simulink model "gm_soc_dvbs2_fpga"  (R2025b)
settings: Solver=VariableStepAuto  StartTime=0.0  StopTime=10.0  RelTol=1e-3
InitFcn:
  | soc_dvbs2_init;
undefined symbols (not defined in the file or in its folder): Add, coefficientsLog, coefficientsSqrt1, coefficientsSqrt2, dataBits, Deinterleaver, designMultirateFIR, noisePow, Shift, Short, soc_dvbs2_designFIRFilter, soc_dvbs2_txPacketBits, syncWord, txDataOut, txFiltCoeff, XData
libraries: simulink x304, hdlsllib x265, dspsigops x15, dsphdlfiltering2 x8, hdlmdlgenlib x6, dsphdlsigops2 x5, commseqgen3 x5, dsphdlmathfun2 x3, hwlogicconnlib x2, whdledac x2, commhdlcrc x2, whdlutilities x1
(part 28 of 36)

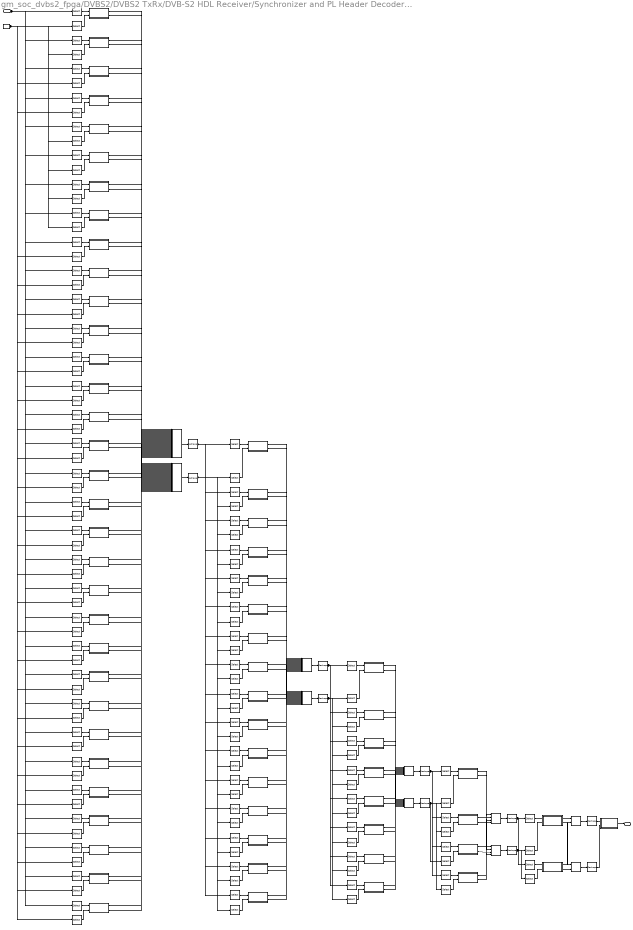
== system gm_soc_dvbs2_fpga/DVBS2/DVBS2 TxRx/DVB-S2 HDL Receiver/Synchronizer and PL Header Decoder/PL Header Recovery/PL Header Decoder/ML Decoder/Get Min Index ==
  dataIn : Inport  OutDataTypeStr=fixdt(1, 25, 15)  PortDimensions=[64]  SampleTime=2.5e-07
  For Each Subsystem1_instance1 : Subsystem
  For Each Subsystem1_instance10 : Subsystem
  For Each Subsystem1_instance11 : Subsystem
  For Each Subsystem1_instance12 : Subsystem
  For Each Subsystem1_instance13 : Subsystem
  For Each Subsystem1_instance14 : Subsystem
  For Each Subsystem1_instance15 : Subsystem
  For Each Subsystem1_instance16 : Subsystem
  For Each Subsystem1_instance2 : Subsystem
  For Each Subsystem1_instance3 : Subsystem
  For Each Subsystem1_instance4 : Subsystem
  For Each Subsystem1_instance5 : Subsystem
  For Each Subsystem1_instance6 : Subsystem
  For Each Subsystem1_instance7 : Subsystem
  For Each Subsystem1_instance8 : Subsystem
  For Each Subsystem1_instance9 : Subsystem
  For Each Subsystem2_instance1 : Subsystem
  For Each Subsystem2_instance2 : Subsystem
  For Each Subsystem2_instance3 : Subsystem
  For Each Subsystem2_instance4 : Subsystem
  For Each Subsystem2_instance5 : Subsystem
  For Each Subsystem2_instance6 : Subsystem
  For Each Subsystem2_instance7 : Subsystem
  For Each Subsystem2_instance8 : Subsystem
  For Each Subsystem3_instance1 : Subsystem
  For Each Subsystem3_instance2 : Subsystem
  For Each Subsystem3_instance3 : Subsystem
  For Each Subsystem3_instance4 : Subsystem
  For Each Subsystem4_instance1 : Subsystem
  For Each Subsystem4_instance2 : Subsystem
  For Each Subsystem5 : Subsystem
  For Each Subsystem_instance1 : Subsystem
  For Each Subsystem_instance10 : Subsystem
  For Each Subsystem_instance11 : Subsystem
  For Each Subsystem_instance12 : Subsystem
  For Each Subsystem_instance13 : Subsystem
  For Each Subsystem_instance14 : Subsystem
  For Each Subsystem_instance15 : Subsystem
  For Each Subsystem_instance16 : Subsystem
  For Each Subsystem_instance17 : Subsystem
  For Each Subsystem_instance18 : Subsystem
  For Each Subsystem_instance19 : Subsystem
  For Each Subsystem_instance2 : Subsystem
  For Each Subsystem_instance20 : Subsystem
  For Each Subsystem_instance21 : Subsystem
  For Each Subsystem_instance22 : Subsystem
  For Each Subsystem_instance23 : Subsystem
  For Each Subsystem_instance24 : Subsystem
  For Each Subsystem_instance25 : Subsystem
  For Each Subsystem_instance26 : Subsystem
  For Each Subsystem_instance27 : Subsystem
  For Each Subsystem_instance28 : Subsystem
  For Each Subsystem_instance29 : Subsystem
  For Each Subsystem_instance3 : Subsystem
  For Each Subsystem_instance30 : Subsystem
  For Each Subsystem_instance31 : Subsystem
  For Each Subsystem_instance32 : Subsystem
  For Each Subsystem_instance4 : Subsystem
  For Each Subsystem_instance5 : Subsystem
  For Each Subsystem_instance6 : Subsystem
  For Each Subsystem_instance7 : Subsystem
  For Each Subsystem_instance8 : Subsystem
  For Each Subsystem_instance9 : Subsystem
  Selector_1 : Selector  InputPortWidth=64  IndexOptions=Index vector (dialog)  Indices=double([1 2])  OutputSizes=1
  Selector_10 : Selector  InputPortWidth=64  IndexOptions=Index vector (dialog)  Indices=double([19 20])  OutputSizes=1
  Selector_101 : Selector  InputPortWidth=64  IndexOptions=Index vector (dialog)  Indices=double([19 20])  OutputSizes=1
  Selector_102 : Selector  InputPortWidth=32  IndexOptions=Index vector (dialog)  Indices=double([19 20])  OutputSizes=1
  Selector_103 : Selector  InputPortWidth=32  IndexOptions=Index vector (dialog)  Indices=double([19 20])  OutputSizes=1
  Selector_11 : Selector  InputPortWidth=64  IndexOptions=Index vector (dialog)  Indices=double([21 22])  OutputSizes=1
  Selector_110 : Selector  InputPortWidth=64  IndexOptions=Index vector (dialog)  Indices=double([1 2])  OutputSizes=1
  Selector_111 : Selector  InputPortWidth=64  IndexOptions=Index vector (dialog)  Indices=double([21 22])  OutputSizes=1
  Selector_112 : Selector  InputPortWidth=32  IndexOptions=Index vector (dialog)  Indices=double([1 2])  OutputSizes=1
  Selector_113 : Selector  InputPortWidth=32  IndexOptions=Index vector (dialog)  Indices=double([21 22])  OutputSizes=1
  Selector_114 : Selector  InputPortWidth=32  IndexOptions=Index vector (dialog)  Indices=double([1 2])  OutputSizes=1
  Selector_115 : Selector  InputPortWidth=32  IndexOptions=Index vector (dialog)  Indices=double([21 22])  OutputSizes=1
  Selector_116 : Selector  InputPortWidth=16  IndexOptions=Index vector (dialog)  Indices=double([1 2])  OutputSizes=1
  Selector_117 : Selector  InputPortWidth=16  IndexOptions=Index vector (dialog)  Indices=double([1 2])  OutputSizes=1
  Selector_118 : Selector  InputPortWidth=8  IndexOptions=Index vector (dialog)  Indices=double([1 2])  OutputSizes=1
  Selector_119 : Selector  InputPortWidth=8  IndexOptions=Index vector (dialog)  Indices=double([1 2])  OutputSizes=1
  Selector_12 : Selector  InputPortWidth=64  IndexOptions=Index vector (dialog)  Indices=double([23 24])  OutputSizes=1
  Selector_120 : Selector  InputPortWidth=4  IndexOptions=Index vector (dialog)  Indices=double([1 2])  OutputSizes=1
  Selector_121 : Selector  InputPortWidth=64  IndexOptions=Index vector (dialog)  Indices=double([23 24])  OutputSizes=1
  Selector_122 : Selector  InputPortWidth=32  IndexOptions=Index vector (dialog)  Indices=double([23 24])  OutputSizes=1
  Selector_123 : Selector  InputPortWidth=32  IndexOptions=Index vector (dialog)  Indices=double([23 24])  OutputSizes=1
  Selector_124 : Selector  InputPortWidth=4  IndexOptions=Index vector (dialog)  Indices=double([1 2])  OutputSizes=1
  Selector_13 : Selector  InputPortWidth=64  IndexOptions=Index vector (dialog)  Indices=double([25 26])  OutputSizes=1
  Selector_131 : Selector  InputPortWidth=64  IndexOptions=Index vector (dialog)  Indices=double([25 26])  OutputSizes=1
  Selector_132 : Selector  InputPortWidth=32  IndexOptions=Index vector (dialog)  Indices=double([25 26])  OutputSizes=1
  Selector_133 : Selector  InputPortWidth=32  IndexOptions=Index vector (dialog)  Indices=double([25 26])  OutputSizes=1
  Selector_14 : Selector  InputPortWidth=64  IndexOptions=Index vector (dialog)  Indices=double([27 28])  OutputSizes=1
  Selector_141 : Selector  InputPortWidth=64  IndexOptions=Index vector (dialog)  Indices=double([27 28])  OutputSizes=1
  Selector_142 : Selector  InputPortWidth=32  IndexOptions=Index vector (dialog)  Indices=double([27 28])  OutputSizes=1
  Selector_143 : Selector  InputPortWidth=32  IndexOptions=Index vector (dialog)  Indices=double([27 28])  OutputSizes=1
  Selector_15 : Selector  InputPortWidth=64  IndexOptions=Index vector (dialog)  Indices=double([29 30])  OutputSizes=1
  Selector_151 : Selector  InputPortWidth=64  IndexOptions=Index vector (dialog)  Indices=double([29 30])  OutputSizes=1
  Selector_152 : Selector  InputPortWidth=32  IndexOptions=Index vector (dialog)  Indices=double([29 30])  OutputSizes=1
  Selector_153 : Selector  InputPortWidth=32  IndexOptions=Index vector (dialog)  Indices=double([29 30])  OutputSizes=1
  Selector_16 : Selector  InputPortWidth=64  IndexOptions=Index vector (dialog)  Indices=double([31 32])  OutputSizes=1
  Selector_161 : Selector  InputPortWidth=64  IndexOptions=Index vector (dialog)  Indices=double([31 32])  OutputSizes=1
  Selector_162 : Selector  InputPortWidth=32  IndexOptions=Index vector (dialog)  Indices=double([31 32])  OutputSizes=1
  Selector_163 : Selector  InputPortWidth=32  IndexOptions=Index vector (dialog)  Indices=double([31 32])  OutputSizes=1
  Selector_17 : Selector  InputPortWidth=64  IndexOptions=Index vector (dialog)  Indices=double([33 34])  OutputSizes=1
  Selector_171 : Selector  InputPortWidth=64  IndexOptions=Index vector (dialog)  Indices=double([33 34])  OutputSizes=1
  Selector_18 : Selector  InputPortWidth=64  IndexOptions=Index vector (dialog)  Indices=double([35 36])  OutputSizes=1
  Selector_181 : Selector  InputPortWidth=64  IndexOptions=Index vector (dialog)  Indices=double([35 36])  OutputSizes=1
  Selector_19 : Selector  InputPortWidth=64  IndexOptions=Index vector (dialog)  Indices=double([37 38])  OutputSizes=1
  Selector_191 : Selector  InputPortWidth=64  IndexOptions=Index vector (dialog)  Indices=double([37 38])  OutputSizes=1
  Selector_2 : Selector  InputPortWidth=64  IndexOptions=Index vector (dialog)  Indices=double([3 4])  OutputSizes=1
  Selector_20 : Selector  InputPortWidth=64  IndexOptions=Index vector (dialog)  Indices=double([39 40])  OutputSizes=1
  Selector_201 : Selector  InputPortWidth=64  IndexOptions=Index vector (dialog)  Indices=double([39 40])  OutputSizes=1
  Selector_21 : Selector  InputPortWidth=64  IndexOptions=Index vector (dialog)  Indices=double([41 42])  OutputSizes=1
  Selector_210 : Selector  InputPortWidth=64  IndexOptions=Index vector (dialog)  Indices=double([3 4])  OutputSizes=1
  Selector_211 : Selector  InputPortWidth=64  IndexOptions=Index vector (dialog)  Indices=double([41 42])  OutputSizes=1
  Selector_212 : Selector  InputPortWidth=32  IndexOptions=Index vector (dialog)  Indices=double([3 4])  OutputSizes=1
  Selector_213 : Selector  InputPortWidth=32  IndexOptions=Index vector (dialog)  Indices=double([3 4])  OutputSizes=1
  Selector_214 : Selector  InputPortWidth=16  IndexOptions=Index vector (dialog)  Indices=double([3 4])  OutputSizes=1
  Selector_215 : Selector  InputPortWidth=16  IndexOptions=Index vector (dialog)  Indices=double([3 4])  OutputSizes=1
  Selector_216 : Selector  InputPortWidth=8  IndexOptions=Index vector (dialog)  Indices=double([3 4])  OutputSizes=1
  Selector_217 : Selector  InputPortWidth=8  IndexOptions=Index vector (dialog)  Indices=double([3 4])  OutputSizes=1
  Selector_218 : Selector  InputPortWidth=4  IndexOptions=Index vector (dialog)  Indices=double([3 4])  OutputSizes=1
  Selector_219 : Selector  InputPortWidth=4  IndexOptions=Index vector (dialog)  Indices=double([3 4])  OutputSizes=1
  Selector_22 : Selector  InputPortWidth=64  IndexOptions=Index vector (dialog)  Indices=double([43 44])  OutputSizes=1
  Selector_221 : Selector  InputPortWidth=64  IndexOptions=Index vector (dialog)  Indices=double([43 44])  OutputSizes=1
  Selector_23 : Selector  InputPortWidth=64  IndexOptions=Index vector (dialog)  Indices=double([45 46])  OutputSizes=1
  Selector_231 : Selector  InputPortWidth=64  IndexOptions=Index vector (dialog)  Indices=double([45 46])  OutputSizes=1
  Selector_24 : Selector  InputPortWidth=64  IndexOptions=Index vector (dialog)  Indices=double([47 48])  OutputSizes=1
  Selector_241 : Selector  InputPortWidth=64  IndexOptions=Index vector (dialog)  Indices=double([47 48])  OutputSizes=1
  Selector_25 : Selector  InputPortWidth=64  IndexOptions=Index vector (dialog)  Indices=double([49 50])  OutputSizes=1
  Selector_251 : Selector  InputPortWidth=64  IndexOptions=Index vector (dialog)  Indices=double([49 50])  OutputSizes=1
  Selector_26 : Selector  InputPortWidth=64  IndexOptions=Index vector (dialog)  Indices=double([51 52])  OutputSizes=1
  Selector_261 : Selector  InputPortWidth=64  IndexOptions=Index vector (dialog)  Indices=double([51 52])  OutputSizes=1
  Selector_27 : Selector  InputPortWidth=64  IndexOptions=Index vector (dialog)  Indices=double([53 54])  OutputSizes=1
  Selector_271 : Selector  InputPortWidth=64  IndexOptions=Index vector (dialog)  Indices=double([53 54])  OutputSizes=1
  Selector_28 : Selector  InputPortWidth=64  IndexOptions=Index vector (dialog)  Indices=double([55 56])  OutputSizes=1
  Selector_281 : Selector  InputPortWidth=64  IndexOptions=Index vector (dialog)  Indices=double([55 56])  OutputSizes=1
  Selector_29 : Selector  InputPortWidth=64  IndexOptions=Index vector (dialog)  Indices=double([57 58])  OutputSizes=1
  Selector_291 : Selector  InputPortWidth=64  IndexOptions=Index vector (dialog)  Indices=double([57 58])  OutputSizes=1
  Selector_3 : Selector  InputPortWidth=64  IndexOptions=Index vector (dialog)  Indices=double([5 6])  OutputSizes=1
  Selector_30 : Selector  InputPortWidth=64  IndexOptions=Index vector (dialog)  Indices=double([59 60])  OutputSizes=1
  Selector_301 : Selector  InputPortWidth=64  IndexOptions=Index vector (dialog)  Indices=double([59 60])  OutputSizes=1
  Selector_31 : Selector  InputPortWidth=64  IndexOptions=Index vector (dialog)  Indices=double([61 62])  OutputSizes=1
  Selector_311 : Selector  InputPortWidth=64  IndexOptions=Index vector (dialog)  Indices=double([61 62])  OutputSizes=1
  Selector_32 : Selector  InputPortWidth=64  IndexOptions=Index vector (dialog)  Indices=double([63 64])  OutputSizes=1
  Selector_321 : Selector  InputPortWidth=64  IndexOptions=Index vector (dialog)  Indices=double([63 64])  OutputSizes=1
  Selector_33 : Selector  InputPortWidth=64  IndexOptions=Index vector (dialog)  Indices=double([5 6])  OutputSizes=1
  Selector_34 : Selector  InputPortWidth=32  IndexOptions=Index vector (dialog)  Indices=double([5 6])  OutputSizes=1
  Selector_35 : Selector  InputPortWidth=32  IndexOptions=Index vector (dialog)  Indices=double([5 6])  OutputSizes=1
  Selector_36 : Selector  InputPortWidth=16  IndexOptions=Index vector (dialog)  Indices=double([5 6])  OutputSizes=1
  Selector_37 : Selector  InputPortWidth=16  IndexOptions=Index vector (dialog)  Indices=double([5 6])  OutputSizes=1
  Selector_38 : Selector  InputPortWidth=8  IndexOptions=Index vector (dialog)  Indices=double([5 6])  OutputSizes=1
  Selector_39 : Selector  InputPortWidth=8  IndexOptions=Index vector (dialog)  Indices=double([5 6])  OutputSizes=1
  Selector_4 : Selector  InputPortWidth=64  IndexOptions=Index vector (dialog)  Indices=double([7 8])  OutputSizes=1
  Selector_41 : Selector  InputPortWidth=64  IndexOptions=Index vector (dialog)  Indices=double([7 8])  OutputSizes=1
  Selector_42 : Selector  InputPortWidth=32  IndexOptions=Index vector (dialog)  Indices=double([7 8])  OutputSizes=1
  Selector_43 : Selector  InputPortWidth=32  IndexOptions=Index vector (dialog)  Indices=double([7 8])  OutputSizes=1
  Selector_44 : Selector  InputPortWidth=16  IndexOptions=Index vector (dialog)  Indices=double([7 8])  OutputSizes=1
  Selector_45 : Selector  InputPortWidth=16  IndexOptions=Index vector (dialog)  Indices=double([7 8])  OutputSizes=1
  Selector_46 : Selector  InputPortWidth=8  IndexOptions=Index vector (dialog)  Indices=double([7 8])  OutputSizes=1
  Selector_47 : Selector  InputPortWidth=8  IndexOptions=Index vector (dialog)  Indices=double([7 8])  OutputSizes=1
  Selector_5 : Selector  InputPortWidth=64  IndexOptions=Index vector (dialog)  Indices=double([9 10])  OutputSizes=1
  Selector_51 : Selector  InputPortWidth=64  IndexOptions=Index vector (dialog)  Indices=double([9 10])  OutputSizes=1
  Selector_52 : Selector  InputPortWidth=32  IndexOptions=Index vector (dialog)  Indices=double([9 10])  OutputSizes=1
  Selector_53 : Selector  InputPortWidth=32  IndexOptions=Index vector (dialog)  Indices=double([9 10])  OutputSizes=1
  Selector_54 : Selector  InputPortWidth=16  IndexOptions=Index vector (dialog)  Indices=double([9 10])  OutputSizes=1
  Selector_55 : Selector  InputPortWidth=16  IndexOptions=Index vector (dialog)  Indices=double([9 10])  OutputSizes=1
  Selector_6 : Selector  InputPortWidth=64  IndexOptions=Index vector (dialog)  Indices=double([11 12])  OutputSizes=1
  Selector_61 : Selector  InputPortWidth=64  IndexOptions=Index vector (dialog)  Indices=double([11 12])  OutputSizes=1
  Selector_62 : Selector  InputPortWidth=32  IndexOptions=Index vector (dialog)  Indices=double([11 12])  OutputSizes=1
  Selector_63 : Selector  InputPortWidth=32  IndexOptions=Index vector (dialog)  Indices=double([11 12])  OutputSizes=1
  Selector_64 : Selector  InputPortWidth=16  IndexOptions=Index vector (dialog)  Indices=double([11 12])  OutputSizes=1
  Selector_65 : Selector  InputPortWidth=16  IndexOptions=Index vector (dialog)  Indices=double([11 12])  OutputSizes=1
  Selector_7 : Selector  InputPortWidth=64  IndexOptions=Index vector (dialog)  Indices=double([13 14])  OutputSizes=1
  Selector_71 : Selector  InputPortWidth=64  IndexOptions=Index vector (dialog)  Indices=double([13 14])  OutputSizes=1
  Selector_72 : Selector  InputPortWidth=32  IndexOptions=Index vector (dialog)  Indices=double([13 14])  OutputSizes=1
  Selector_73 : Selector  InputPortWidth=32  IndexOptions=Index vector (dialog)  Indices=double([13 14])  OutputSizes=1
  Selector_74 : Selector  InputPortWidth=16  IndexOptions=Index vector (dialog)  Indices=double([13 14])  OutputSizes=1
  Selector_75 : Selector  InputPortWidth=16  IndexOptions=Index vector (dialog)  Indices=double([13 14])  OutputSizes=1
  Selector_8 : Selector  InputPortWidth=64  IndexOptions=Index vector (dialog)  Indices=double([15 16])  OutputSizes=1
  Selector_81 : Selector  InputPortWidth=64  IndexOptions=Index vector (dialog)  Indices=double([15 16])  OutputSizes=1
  Selector_82 : Selector  InputPortWidth=32  IndexOptions=Index vector (dialog)  Indices=double([15 16])  OutputSizes=1
  Selector_83 : Selector  InputPortWidth=32  IndexOptions=Index vector (dialog)  Indices=double([15 16])  OutputSizes=1
  Selector_84 : Selector  InputPortWidth=16  IndexOptions=Index vector (dialog)  Indices=double([15 16])  OutputSizes=1
  Selector_85 : Selector  InputPortWidth=16  IndexOptions=Index vector (dialog)  Indices=double([15 16])  OutputSizes=1
  Selector_9 : Selector  InputPortWidth=64  IndexOptions=Index vector (dialog)  Indices=double([17 18])  OutputSizes=1
  Selector_91 : Selector  InputPortWidth=64  IndexOptions=Index vector (dialog)  Indices=double([17 18])  OutputSizes=1
  Selector_92 : Selector  InputPortWidth=32  IndexOptions=Index vector (dialog)  Indices=double([17 18])  OutputSizes=1
  Selector_93 : Selector  InputPortWidth=32  IndexOptions=Index vector (dialog)  Indices=double([17 18])  OutputSizes=1
  concatenate : Concatenate  NumInputs=32
  concatenate1 : Concatenate  NumInputs=32
  concatenate2 : Concatenate  NumInputs=16
  concatenate3 : Concatenate  NumInputs=16
  concatenate4 : Concatenate  NumInputs=8
  concatenate5 : Concatenate  NumInputs=8
  concatenate6 : Concatenate  NumInputs=4
  concatenate7 : Concatenate  NumInputs=4
  concatenate8 : Concatenate
  concatenate9 : Concatenate
  indices : Constant  Value=(0:63).'  OutDataTypeStr=fixdt(0,6,0)  SampleTime=-1
  t{,1..9} (10 alike) : Reshape
  out : Outport  SampleTime=2.5e-07
  wires:
  For Each Subsystem5/1(idxOut) -> out/1
  Selector_75/1 -> For Each Subsystem2_instance7/2(idxIn)
  Selector_39/1 -> For Each Subsystem3_instance3/2(idxIn)
  indices/1 -> Selector_311/1, Selector_271/1, Selector_261/1, Selector_251/1, Selector_241/1, Selector_231/1, Selector_211/1, Selector_181/1, Selector_171/1, Selector_131/1, Selector_101/1, Selector_81/1, Selector_61/1, Selector_41/1, Selector_33/1, Selector_210/1, Selector_110/1, Selector_281/1, Selector_161/1, Selector_301/1, Selector_91/1, Selector_151/1, Selector_191/1, Selector_291/1, Selector_121/1, Selector_321/1, Selector_51/1, Selector_111/1, Selector_221/1, Selector_201/1, Selector_71/1, Selector_141/1
  For Each Subsystem2_instance5/1(ValueOut) -> concatenate4/5
  For Each Subsystem2_instance6/1(ValueOut) -> concatenate4/6
  Selector_191/1 -> For Each Subsystem_instance19/2(idxIn)
  For Each Subsystem2_instance3/1(ValueOut) -> concatenate4/3
  Selector_35/1 -> For Each Subsystem1_instance3/2(idxIn)
  For Each Subsystem4_instance2/2(idxOut) -> concatenate9/2
  For Each Subsystem2_instance7/2(idxOut) -> concatenate5/7
  For Each Subsystem3_instance4/1(ValueOut) -> concatenate6/4
  For Each Subsystem2_instance1/2(idxOut) -> concatenate5/1
  For Each Subsystem_instance17/1(ValueOut) -> concatenate/17
  concatenate9/1 -> t9/1
  Selector_118/1 -> For Each Subsystem3_instance1/1(valueIn)
  Selector_16/1 -> For Each Subsystem_instance16/1(valueIn)
  For Each Subsystem3_instance2/2(idxOut) -> concatenate7/2
  Selector_1/1 -> For Each Subsystem_instance1/1(valueIn)
  Selector_74/1 -> For Each Subsystem2_instance7/1(valueIn)
  For Each Subsystem1_instance16/2(idxOut) -> concatenate3/16
  Selector_53/1 -> For Each Subsystem1_instance5/2(idxIn)
  Selector_291/1 -> For Each Subsystem_instance29/2(idxIn)
  For Each Subsystem2_instance3/2(idxOut) -> concatenate5/3
  Selector_17/1 -> For Each Subsystem_instance17/1(valueIn)
  concatenate7/1 -> t7/1
  For Each Subsystem4_instance2/1(ValueOut) -> concatenate8/2
  Selector_55/1 -> For Each Subsystem2_instance5/2(idxIn)
  t1/1 -> Selector_163/1, Selector_153/1, Selector_143/1, Selector_123/1, Selector_103/1, Selector_93/1, Selector_83/1, Selector_73/1, Selector_63/1, Selector_53/1, Selector_213/1, Selector_114/1, Selector_133/1, Selector_115/1, Selector_35/1, Selector_43/1
  For Each Subsystem_instance10/2(idxOut) -> concatenate1/10
  For Each Subsystem_instance16/2(idxOut) -> concatenate1/16
  Selector_116/1 -> For Each Subsystem2_instance1/1(valueIn)
  For Each Subsystem2_instance6/2(idxOut) -> concatenate5/6
  For Each Subsystem3_instance3/1(ValueOut) -> concatenate6/3
  Selector_201/1 -> For Each Subsystem_instance20/2(idxIn)
  For Each Subsystem4_instance1/2(idxOut) -> concatenate9/1
  For Each Subsystem2_instance8/1(ValueOut) -> concatenate4/8
  For Each Subsystem_instance28/2(idxOut) -> concatenate1/28
  Selector_20/1 -> For Each Subsystem_instance20/1(valueIn)
  For Each Subsystem3_instance3/2(idxOut) -> concatenate7/3
  Selector_171/1 -> For Each Subsystem_instance17/2(idxIn)
  For Each Subsystem4_instance1/1(ValueOut) -> concatenate8/1
  Selector_219/1 -> For Each Subsystem4_instance2/2(idxIn)
  For Each Subsystem_instance28/1(ValueOut) -> concatenate/28
  For Each Subsystem2_instance8/2(idxOut) -> concatenate5/8
  concatenate8/1 -> t8/1
  Selector_214/1 -> For Each Subsystem2_instance2/1(valueIn)
  Selector_13/1 -> For Each Subsystem_instance13/1(valueIn)
  Selector_124/1 -> For Each Subsystem4_instance1/2(idxIn)
  Selector_4/1 -> For Each Subsystem_instance4/1(valueIn)
  Selector_218/1 -> For Each Subsystem4_instance2/1(valueIn)
  Selector_45/1 -> For Each Subsystem2_instance4/2(idxIn)
  For Each Subsystem_instance9/1(ValueOut) -> concatenate/9
  For Each Subsystem_instance30/1(ValueOut) -> concatenate/30
  t2/1 -> Selector_84/1, Selector_74/1, Selector_44/1, Selector_36/1, Selector_116/1, Selector_54/1, Selector_64/1, Selector_214/1
  t5/1 -> Selector_47/1, Selector_39/1, Selector_217/1, Selector_119/1
  For Each Subsystem3_instance1/2(idxOut) -> concatenate7/1
  Selector_120/1 -> For Each Subsystem4_instance1/1(valueIn)
  Selector_133/1 -> For Each Subsystem1_instance13/2(idxIn)
  Selector_85/1 -> For Each Subsystem2_instance8/2(idxIn)
  For Each Subsystem3_instance4/2(idxOut) -> concatenate7/4
  Selector_65/1 -> For Each Subsystem2_instance6/2(idxIn)
  Selector_217/1 -> For Each Subsystem3_instance2/2(idxIn)
  Selector_19/1 -> For Each Subsystem_instance19/1(valueIn)
  For Each Subsystem1_instance11/2(idxOut) -> concatenate3/11
  For Each Subsystem2_instance2/2(idxOut) -> concatenate5/2
  For Each Subsystem1_instance2/2(idxOut) -> concatenate3/2
  Selector_216/1 -> For Each Subsystem3_instance2/1(valueIn)
  For Each Subsystem3_instance2/1(ValueOut) -> concatenate6/2
  For Each Subsystem3_instance1/1(ValueOut) -> concatenate6/1
  Selector_44/1 -> For Each Subsystem2_instance4/1(valueIn)
  Selector_162/1 -> For Each Subsystem1_instance16/1(valueIn)
  concatenate6/1 -> t6/1
  Selector_47/1 -> For Each Subsystem3_instance4/2(idxIn)
  Selector_210/1 -> For Each Subsystem_instance2/2(idxIn)
  For Each Subsystem_instance18/2(idxOut) -> concatenate1/18
  Selector_38/1 -> For Each Subsystem3_instance3/1(valueIn)
  For Each Subsystem_instance32/2(idxOut) -> concatenate1/32
  For Each Subsystem_instance29/2(idxOut) -> concatenate1/29
  Selector_119/1 -> For Each Subsystem3_instance1/2(idxIn)
  Selector_112/1 -> For Each Subsystem1_instance1/1(valueIn)
  Selector_46/1 -> For Each Subsystem3_instance4/1(valueIn)
  dataIn/1 -> Selector_30/1, Selector_23/1, Selector_22/1, Selector_20/1, Selector_17/1, Selector_10/1, Selector_18/1, Selector_9/1, Selector_7/1, Selector_3/1, Selector_14/1, Selector_24/1, Selector_5/1, Selector_4/1, Selector_25/1, Selector_19/1, Selector_13/1, Selector_11/1, Selector_15/1, Selector_28/1, Selector_31/1, Selector_29/1, Selector_26/1, Selector_21/1, Selector_2/1, Selector_16/1, Selector_12/1, Selector_27/1, Selector_8/1, Selector_32/1, Selector_1/1, Selector_6/1
  For Each Subsystem_instance31/1(ValueOut) -> concatenate/31
  For Each Subsystem1_instance8/2(idxOut) -> concatenate3/8
  For Each Subsystem2_instance5/2(idxOut) -> concatenate5/5
  For Each Subsystem2_instance4/2(idxOut) -> concatenate5/4
  concatenate5/1 -> t5/1
  For Each Subsystem2_instance7/1(ValueOut) -> concatenate4/7
  For Each Subsystem_instance21/1(ValueOut) -> concatenate/21
  For Each Subsystem_instance18/1(ValueOut) -> concatenate/18
  Selector_93/1 -> For Each Subsystem1_instance9/2(idxIn)
  For Each Subsystem2_instance4/1(ValueOut) -> concatenate4/4
  For Each Subsystem2_instance2/1(ValueOut) -> concatenate4/2
  For Each Subsystem2_instance1/1(ValueOut) -> concatenate4/1
  Selector_123/1 -> For Each Subsystem1_instance12/2(idxIn)
  t7/1 -> Selector_219/1, Selector_124/1
  Selector_92/1 -> For Each Subsystem1_instance9/1(valueIn)
  For Each Subsystem_instance23/2(idxOut) -> concatenate1/23
  concatenate4/1 -> t4/1
  Selector_213/1 -> For Each Subsystem1_instance2/2(idxIn)
  Selector_37/1 -> For Each Subsystem2_instance3/2(idxIn)
  Selector_84/1 -> For Each Subsystem2_instance8/1(valueIn)
  Selector_215/1 -> For Each Subsystem2_instance2/2(idxIn)
  For Each Subsystem1_instance3/2(idxOut) -> concatenate3/3
  For Each Subsystem_instance3/2(idxOut) -> concatenate1/3
  Selector_117/1 -> For Each Subsystem2_instance1/2(idxIn)
  Selector_64/1 -> For Each Subsystem2_instance6/1(valueIn)
  Selector_321/1 -> For Each Subsystem_instance32/2(idxIn)
  Selector_54/1 -> For Each Subsystem2_instance5/1(valueIn)
  Selector_36/1 -> For Each Subsystem2_instance3/1(valueIn)
  Selector_281/1 -> For Each Subsystem_instance28/2(idxIn)
  For Each Subsystem_instance9/2(idxOut) -> concatenate1/9
  For Each Subsystem1_instance15/2(idxOut) -> concatenate3/15
  Selector_34/1 -> For Each Subsystem1_instance3/1(valueIn)
  For Each Subsystem1_instance14/2(idxOut) -> concatenate3/14
  Selector_12/1 -> For Each Subsystem_instance12/1(valueIn)
  For Each Subsystem1_instance13/2(idxOut) -> concatenate3/13
  For Each Subsystem1_instance12/2(idxOut) -> concatenate3/12
  Selector_271/1 -> For Each Subsystem_instance27/2(idxIn)
  For Each Subsystem1_instance10/2(idxOut) -> concatenate3/10
  concatenate/1 -> t/1
  For Each Subsystem1_instance9/2(idxOut) -> concatenate3/9
  Selector_143/1 -> For Each Subsystem1_instance14/2(idxIn)
  For Each Subsystem1_instance7/2(idxOut) -> concatenate3/7
  For Each Subsystem_instance4/1(ValueOut) -> concatenate/4
  For Each Subsystem_instance10/1(ValueOut) -> concatenate/10
  Selector_11/1 -> For Each Subsystem_instance11/1(valueIn)
  Selector_261/1 -> For Each Subsystem_instance26/2(idxIn)
  Selector_102/1 -> For Each Subsystem1_instance10/1(valueIn)
  For Each Subsystem1_instance9/1(ValueOut) -> concatenate2/9
  For Each Subsystem1_instance6/2(idxOut) -> concatenate3/6
  For Each Subsystem1_instance5/2(idxOut) -> concatenate3/5
  For Each Subsystem1_instance4/2(idxOut) -> concatenate3/4
  For Each Subsystem_instance4/2(idxOut) -> concatenate1/4
  For Each Subsystem1_instance1/2(idxOut) -> concatenate3/1
  concatenate3/1 -> t3/1
  For Each Subsystem1_instance16/1(ValueOut) -> concatenate2/16
  For Each Subsystem1_instance15/1(ValueOut) -> concatenate2/15
  t/1 -> Selector_152/1, Selector_113/1, Selector_82/1, Selector_42/1, Selector_34/1, Selector_72/1, Selector_212/1, Selector_52/1, Selector_132/1, Selector_122/1, Selector_112/1, Selector_92/1, Selector_142/1, Selector_62/1, Selector_162/1, Selector_102/1
  Selector_22/1 -> For Each Subsystem_instance22/1(valueIn)
  For Each Subsystem1_instance14/1(ValueOut) -> concatenate2/14
  For Each Subsystem1_instance13/1(ValueOut) -> concatenate2/13
  For Each Subsystem1_instance12/1(ValueOut) -> concatenate2/12
  For Each Subsystem1_instance11/1(ValueOut) -> concatenate2/11
  Selector_5/1 -> For Each Subsystem_instance5/1(valueIn)
  For Each Subsystem1_instance10/1(ValueOut) -> concatenate2/10
  For Each Subsystem1_instance8/1(ValueOut) -> concatenate2/8
  For Each Subsystem1_instance4/1(ValueOut) -> concatenate2/4
  For Each Subsystem1_instance7/1(ValueOut) -> concatenate2/7
  For Each Subsystem1_instance6/1(ValueOut) -> concatenate2/6
  For Each Subsystem1_instance5/1(ValueOut) -> concatenate2/5
  For Each Subsystem1_instance3/1(ValueOut) -> concatenate2/3
  Selector_81/1 -> For Each Subsystem_instance8/2(idxIn)
  t6/1 -> Selector_120/1, Selector_218/1
  For Each Subsystem1_instance2/1(ValueOut) -> concatenate2/2
  For Each Subsystem1_instance1/1(ValueOut) -> concatenate2/1
  For Each Subsystem_instance3/1(ValueOut) -> concatenate/3
  concatenate2/1 -> t2/1
  Selector_163/1 -> For Each Subsystem1_instance16/2(idxIn)
  Selector_21/1 -> For Each Subsystem_instance21/1(valueIn)
  Selector_153/1 -> For Each Subsystem1_instance15/2(idxIn)
  Selector_115/1 -> For Each Subsystem1_instance11/2(idxIn)
  Selector_241/1 -> For Each Subsystem_instance24/2(idxIn)
  Selector_122/1 -> For Each Subsystem1_instance12/1(valueIn)
  Selector_103/1 -> For Each Subsystem1_instance10/2(idxIn)
  For Each Subsystem_instance15/2(idxOut) -> concatenate1/15
  Selector_83/1 -> For Each Subsystem1_instance8/2(idxIn)
  Selector_73/1 -> For Each Subsystem1_instance7/2(idxIn)
  For Each Subsystem_instance12/2(idxOut) -> concatenate1/12
  Selector_63/1 -> For Each Subsystem1_instance6/2(idxIn)
  Selector_43/1 -> For Each Subsystem1_instance4/2(idxIn)
  For Each Subsystem_instance11/2(idxOut) -> concatenate1/11
  Selector_114/1 -> For Each Subsystem1_instance1/2(idxIn)
  Selector_152/1 -> For Each Subsystem1_instance15/1(valueIn)
  For Each Subsystem_instance7/2(idxOut) -> concatenate1/7
  Selector_142/1 -> For Each Subsystem1_instance14/1(valueIn)
  For Each Subsystem_instance23/1(ValueOut) -> concatenate/23
  Selector_51/1 -> For Each Subsystem_instance5/2(idxIn)
  Selector_132/1 -> For Each Subsystem1_instance13/1(valueIn)
  Selector_113/1 -> For Each Subsystem1_instance11/1(valueIn)
  For Each Subsystem_instance1/1(ValueOut) -> concatenate/1
  Selector_82/1 -> For Each Subsystem1_instance8/1(valueIn)
  Selector_121/1 -> For Each Subsystem_instance12/2(idxIn)
  Selector_72/1 -> For Each Subsystem1_instance7/1(valueIn)
  Selector_141/1 -> For Each Subsystem_instance14/2(idxIn)
  Selector_62/1 -> For Each Subsystem1_instance6/1(valueIn)
  Selector_131/1 -> For Each Subsystem_instance13/2(idxIn)
  Selector_52/1 -> For Each Subsystem1_instance5/1(valueIn)
  Selector_32/1 -> For Each Subsystem_instance32/1(valueIn)
  Selector_42/1 -> For Each Subsystem1_instance4/1(valueIn)
  Selector_212/1 -> For Each Subsystem1_instance2/1(valueIn)
  For Each Subsystem_instance31/2(idxOut) -> concatenate1/31
  For Each Subsystem_instance30/2(idxOut) -> concatenate1/30
  For Each Subsystem_instance27/2(idxOut) -> concatenate1/27
  For Each Subsystem_instance26/2(idxOut) -> concatenate1/26
  For Each Subsystem_instance25/2(idxOut) -> concatenate1/25
  For Each Subsystem_instance24/2(idxOut) -> concatenate1/24
  For Each Subsystem_instance22/2(idxOut) -> concatenate1/22
  For Each Subsystem_instance1/2(idxOut) -> concatenate1/1
  concatenate1/1 -> t1/1
  For Each Subsystem_instance21/2(idxOut) -> concatenate1/21
  t9/1 -> For Each Subsystem5/2(idxIn)
  For Each Subsystem_instance17/2(idxOut) -> concatenate1/17
  For Each Subsystem_instance20/2(idxOut) -> concatenate1/20
  Selector_26/1 -> For Each Subsystem_instance26/1(valueIn)
  For Each Subsystem_instance19/2(idxOut) -> concatenate1/19
  For Each Subsystem_instance14/2(idxOut) -> concatenate1/14
  For Each Subsystem_instance13/2(idxOut) -> concatenate1/13
  For Each Subsystem_instance8/2(idxOut) -> concatenate1/8
  For Each Subsystem_instance6/2(idxOut) -> concatenate1/6
  For Each Subsystem_instance5/2(idxOut) -> concatenate1/5
  Selector_31/1 -> For Each Subsystem_instance31/1(valueIn)
  For Each Subsystem_instance19/1(ValueOut) -> concatenate/19
  For Each Subsystem_instance2/2(idxOut) -> concatenate1/2
  For Each Subsystem_instance24/1(ValueOut) -> concatenate/24
  For Each Subsystem_instance27/1(ValueOut) -> concatenate/27
  For Each Subsystem_instance32/1(ValueOut) -> concatenate/32
  For Each Subsystem_instance29/1(ValueOut) -> concatenate/29
  For Each Subsystem_instance26/1(ValueOut) -> concatenate/26
  For Each Subsystem_instance25/1(ValueOut) -> concatenate/25
  Selector_10/1 -> For Each Subsystem_instance10/1(valueIn)
  Selector_15/1 -> For Each Subsystem_instance15/1(valueIn)
  Selector_181/1 -> For Each Subsystem_instance18/2(idxIn)
  Selector_27/1 -> For Each Subsystem_instance27/1(valueIn)
  For Each Subsystem_instance22/1(ValueOut) -> concatenate/22
  Selector_6/1 -> For Each Subsystem_instance6/1(valueIn)
  For Each Subsystem_instance20/1(ValueOut) -> concatenate/20
  For Each Subsystem_instance16/1(ValueOut) -> concatenate/16
  Selector_9/1 -> For Each Subsystem_instance9/1(valueIn)
  t3/1 -> Selector_75/1, Selector_65/1, Selector_37/1, Selector_117/1, Selector_215/1, Selector_55/1, Selector_85/1, Selector_45/1
  For Each Subsystem_instance15/1(ValueOut) -> concatenate/15
  Selector_101/1 -> For Each Subsystem_instance10/2(idxIn)
  For Each Subsystem_instance14/1(ValueOut) -> concatenate/14
  For Each Subsystem_instance7/1(ValueOut) -> concatenate/7
  For Each Subsystem_instance13/1(ValueOut) -> concatenate/13
  For Each Subsystem_instance12/1(ValueOut) -> concatenate/12
  For Each Subsystem_instance11/1(ValueOut) -> concatenate/11
  For Each Subsystem_instance8/1(ValueOut) -> concatenate/8
  For Each Subsystem_instance6/1(ValueOut) -> concatenate/6
  For Each Subsystem_instance5/1(ValueOut) -> concatenate/5
  For Each Subsystem_instance2/1(ValueOut) -> concatenate/2
  Selector_311/1 -> For Each Subsystem_instance31/2(idxIn)
  Selector_211/1 -> For Each Subsystem_instance21/2(idxIn)
  Selector_301/1 -> For Each Subsystem_instance30/2(idxIn)
  Selector_251/1 -> For Each Subsystem_instance25/2(idxIn)
  Selector_18/1 -> For Each Subsystem_instance18/1(valueIn)
  Selector_231/1 -> For Each Subsystem_instance23/2(idxIn)
  Selector_221/1 -> For Each Subsystem_instance22/2(idxIn)
  t4/1 -> Selector_46/1, Selector_38/1, Selector_118/1, Selector_216/1
  Selector_161/1 -> For Each Subsystem_instance16/2(idxIn)
  Selector_151/1 -> For Each Subsystem_instance15/2(idxIn)
  t8/1 -> For Each Subsystem5/1(valueIn)
  Selector_23/1 -> For Each Subsystem_instance23/1(valueIn)
  Selector_111/1 -> For Each Subsystem_instance11/2(idxIn)
  Selector_91/1 -> For Each Subsystem_instance9/2(idxIn)
  Selector_71/1 -> For Each Subsystem_instance7/2(idxIn)
  Selector_61/1 -> For Each Subsystem_instance6/2(idxIn)
  Selector_41/1 -> For Each Subsystem_instance4/2(idxIn)
  Selector_33/1 -> For Each Subsystem_instance3/2(idxIn)
  Selector_110/1 -> For Each Subsystem_instance1/2(idxIn)
  Selector_30/1 -> For Each Subsystem_instance30/1(valueIn)
  Selector_29/1 -> For Each Subsystem_instance29/1(valueIn)
  Selector_28/1 -> For Each Subsystem_instance28/1(valueIn)
  Selector_25/1 -> For Each Subsystem_instance25/1(valueIn)
  Selector_24/1 -> For Each Subsystem_instance24/1(valueIn)
  Selector_14/1 -> For Each Subsystem_instance14/1(valueIn)
  Selector_8/1 -> For Each Subsystem_instance8/1(valueIn)
  Selector_7/1 -> For Each Subsystem_instance7/1(valueIn)
  Selector_3/1 -> For Each Subsystem_instance3/1(valueIn)
  Selector_2/1 -> For Each Subsystem_instance2/1(valueIn)
